simulink model "SWC_TRSP"  (R2020a)
settings: Solver=FixedStepDiscrete  StartTime=0.0  StopTime=0.15  FixedStep=0.0001  RelTol=1e-3
values from neighbouring files (symbols this model uses):
  CAL_TRSP_18VHSVoltCountTrh_s16 = 0.0    [SWC_TRSP_DataDictionary.sldd]
  CAL_TRSP_18VHSVoltDebTrh_s16 = 0.0    [SWC_TRSP_DataDictionary.sldd]
  CAL_TRSP_18VHSVoltErrRst_b = 0.0    [SWC_TRSP_DataDictionary.sldd]
  CAL_TRSP_18VHSVoltHiLim_u16 = 0.0    [SWC_TRSP_DataDictionary.sldd]
  CAL_TRSP_18VHSVoltLoLim_u16 = 0.0    [SWC_TRSP_DataDictionary.sldd]
  CAL_TRSP_1V8CPLDVoltCountTrh_s16 = 0.0    [SWC_TRSP_DataDictionary.sldd]
  CAL_TRSP_1V8CPLDVoltDebTrh_s16 = 0.0    [SWC_TRSP_DataDictionary.sldd]
  CAL_TRSP_1V8CPLDVoltErrRst_b = 0.0    [SWC_TRSP_DataDictionary.sldd]
  CAL_TRSP_1V8CPLDVoltHiLim_u16 = 0.0    [SWC_TRSP_DataDictionary.sldd]
  CAL_TRSP_1V8CPLDVoltLoLim_u16 = 0.0    [SWC_TRSP_DataDictionary.sldd]
  CAL_TRSP_3V3CPLDVoltCountTrh_s16 = 0.0    [SWC_TRSP_DataDictionary.sldd]
  CAL_TRSP_3V3CPLDVoltDebTrh_s16 = 0.0    [SWC_TRSP_DataDictionary.sldd]
  CAL_TRSP_3V3CPLDVoltErrRst_b = 0.0    [SWC_TRSP_DataDictionary.sldd]
  CAL_TRSP_3V3CPLDVoltHiLim_u16 = 0.0    [SWC_TRSP_DataDictionary.sldd]
  CAL_TRSP_3V3CPLDVoltLoLim_u16 = 0.0    [SWC_TRSP_DataDictionary.sldd]
  CAL_TRSP_AgTimecompCtl_u8 = 0.0    [SWC_TRSP_DataDictionary.sldd]
  CAL_TRSP_CurrRngCountTrh_s16 = 0.0    [SWC_TRSP_DataDictionary.sldd]
  CAL_TRSP_CurrRngDebTrh_s16 = 0.0    [SWC_TRSP_DataDictionary.sldd]
  CAL_TRSP_CurrRngErrRst_b = 0.0    [SWC_TRSP_DataDictionary.sldd]
  CAL_TRSP_CurrSumCountTrh_s16 = 0.0    [SWC_TRSP_DataDictionary.sldd]
  CAL_TRSP_CurrSumDebTrh_s16 = 0.0    [SWC_TRSP_DataDictionary.sldd]
  CAL_TRSP_CurrSumErrRst_b = 0.0    [SWC_TRSP_DataDictionary.sldd]
  CAL_TRSP_CurrSumLim_f32 = 0.0    [SWC_TRSP_DataDictionary.sldd]
  CAL_TRSP_Diff_UBR_SBCLim_f32 = 0.0    [SWC_TRSP_DataDictionary.sldd]
  CAL_TRSP_flgChangPha_b = 0.0    [SWC_TRSP_DataDictionary.sldd]
  CAL_TRSP_iPhasSensVoltCountTrh_s16 = 0.0    [SWC_TRSP_DataDictionary.sldd]
  CAL_TRSP_iPhasSensVoltDebTrh_s16 = 0.0    [SWC_TRSP_DataDictionary.sldd]
  CAL_TRSP_iPhasSensVoltErrRst_b = 0.0    [SWC_TRSP_DataDictionary.sldd]
  CAL_TRSP_iPhasSensVoltHiLim_u16 = 0.0    [SWC_TRSP_DataDictionary.sldd]
  CAL_TRSP_iPhasSensVoltLoLim_u16 = 0.0    [SWC_TRSP_DataDictionary.sldd]
  CAL_TRSP_iPhaUOffset_f32 = 0.0    [SWC_TRSP_DataDictionary.sldd]
  CAL_TRSP_iPhaVOffset_f32 = 0.0    [SWC_TRSP_DataDictionary.sldd]
  CAL_TRSP_iPhaWOffset_f32 = 0.0    [SWC_TRSP_DataDictionary.sldd]
  CAL_TRSP_iUCnvFac_f32 = 0.0    [SWC_TRSP_DataDictionary.sldd]
  CAL_TRSP_iVCnvFac_f32 = 0.0    [SWC_TRSP_DataDictionary.sldd]
  CAL_TRSP_iWCnvFac_f32 = 0.0    [SWC_TRSP_DataDictionary.sldd]
  CAL_TRSP_OfstErrRst_b = 0.0    [SWC_TRSP_DataDictionary.sldd]
  CAL_TRSP_OfstRngHiLim_f32 = 0.0    [SWC_TRSP_DataDictionary.sldd]
  CAL_TRSP_OfstRngLoLim_f32 = 0.0    [SWC_TRSP_DataDictionary.sldd]
  CAL_TRSP_ReqTrqCountTrh_s16 = 0.0    [SWC_TRSP_DataDictionary.sldd]
  CAL_TRSP_ReqTrqDebTrh_s16 = 0.0    [SWC_TRSP_DataDictionary.sldd]
  CAL_TRSP_ReqTrqErrRst_b = 0.0    [SWC_TRSP_DataDictionary.sldd]
  CAL_TRSP_ReqTrqHiLim_f32 = 0.0    [SWC_TRSP_DataDictionary.sldd]
  CAL_TRSP_ReqTrqLoLim_f32 = 0.0    [SWC_TRSP_DataDictionary.sldd]
  CAL_TRSP_RslvExciCountTrh_s16 = 0.0    [SWC_TRSP_DataDictionary.sldd]
  CAL_TRSP_RslvExciDebTrh_s16 = 0.0    [SWC_TRSP_DataDictionary.sldd]
  CAL_TRSP_RslvExciErrRst_b = 0.0    [SWC_TRSP_DataDictionary.sldd]
  CAL_TRSP_RslvMaxSele_u8 = 0.0    [SWC_TRSP_DataDictionary.sldd]
  CAL_TRSP_RslvMinSele_u8 = 0.0    [SWC_TRSP_DataDictionary.sldd]
  CAL_TRSP_RslvRngCosNHiLim_u16 = 0.0    [SWC_TRSP_DataDictionary.sldd]
  CAL_TRSP_RslvRngCosNLoLim_u16 = 0.0    [SWC_TRSP_DataDictionary.sldd]
  CAL_TRSP_RslvRngCosPHiLim_u16 = 0.0    [SWC_TRSP_DataDictionary.sldd]
  CAL_TRSP_RslvRngCosPLoLim_u16 = 0.0    [SWC_TRSP_DataDictionary.sldd]
  CAL_TRSP_RslvRngCountTrh_s16 = 0.0    [SWC_TRSP_DataDictionary.sldd]
  CAL_TRSP_RslvRngDebTrh_s16 = 0.0    [SWC_TRSP_DataDictionary.sldd]
  CAL_TRSP_RslvRngErrRst_b = 0.0    [SWC_TRSP_DataDictionary.sldd]
  CAL_TRSP_RslvRngExciHiLim_u16 = 0.0    [SWC_TRSP_DataDictionary.sldd]
  CAL_TRSP_RslvRngExciLoLim_u16 = 0.0    [SWC_TRSP_DataDictionary.sldd]
  CAL_TRSP_RslvRngSinNHiLim_u16 = 0.0    [SWC_TRSP_DataDictionary.sldd]
  CAL_TRSP_RslvRngSinNLoLim_u16 = 0.0    [SWC_TRSP_DataDictionary.sldd]
  CAL_TRSP_RslvRngSinPHiLim_u16 = 0.0    [SWC_TRSP_DataDictionary.sldd]
  CAL_TRSP_RslvRngSinPLoLim_u16 = 0.0    [SWC_TRSP_DataDictionary.sldd]
  CAL_TRSP_RslvSensVoltCountTrh_s16 = 0.0    [SWC_TRSP_DataDictionary.sldd]
  CAL_TRSP_RslvSensVoltDebTrh_s16 = 0.0    [SWC_TRSP_DataDictionary.sldd]
  CAL_TRSP_RslvSensVoltErrRst_b = 0.0    [SWC_TRSP_DataDictionary.sldd]
  CAL_TRSP_RslvSensVoltHiLim_u16 = 0.0    [SWC_TRSP_DataDictionary.sldd]
  CAL_TRSP_RslvSensVoltLoLim_u16 = 0.0    [SWC_TRSP_DataDictionary.sldd]
  CAL_TRSP_RslvSqrtCountTrh_s16 = 0.0    [SWC_TRSP_DataDictionary.sldd]
  CAL_TRSP_RslvSqrtDebTrh_s16 = 0.0    [SWC_TRSP_DataDictionary.sldd]
  CAL_TRSP_RslvSqrtErrRst_b = 0.0    [SWC_TRSP_DataDictionary.sldd]
  CAL_TRSP_RslvSqrtHiLim_u16 = 0.0    [SWC_TRSP_DataDictionary.sldd]
  CAL_TRSP_RslvSqrtLoLim_u16 = 0.0    [SWC_TRSP_DataDictionary.sldd]
  CAL_TRSP_SpeedCtlMode_u8 = 0.0    [SWC_TRSP_DataDictionary.sldd]
  CAL_TRSP_TorqueCtlMode_u8 = 0.0    [SWC_TRSP_DataDictionary.sldd]
  CAL_TRSP_UB_SBCCnvFac_f32 = 0.0    [SWC_TRSP_DataDictionary.sldd]
  CAL_TRSP_UBRVoltCountTrh_s16 = 0.0    [SWC_TRSP_DataDictionary.sldd]
  CAL_TRSP_UBRVoltDebTrh_s16 = 0.0    [SWC_TRSP_DataDictionary.sldd]
  CAL_TRSP_UBRVoltErrRst_b = 0.0    [SWC_TRSP_DataDictionary.sldd]
  CAL_TRSP_UBRWIDECnvFac_f32 = 0.0    [SWC_TRSP_DataDictionary.sldd]
  CAL_TRSP_UCurrRngHiLim_f32 = 0.0    [SWC_TRSP_DataDictionary.sldd]
  CAL_TRSP_UCurrRngLoLim_f32 = 0.0    [SWC_TRSP_DataDictionary.sldd]
  CAL_TRSP_VCurrRngHiLim_f32 = 0.0    [SWC_TRSP_DataDictionary.sldd]
  CAL_TRSP_VCurrRngLoLim_f32 = 0.0    [SWC_TRSP_DataDictionary.sldd]
  CAL_TRSP_WCurrRngHiLim_f32 = 0.0    [SWC_TRSP_DataDictionary.sldd]
  CAL_TRSP_WCurrRngLoLim_f32 = 0.0    [SWC_TRSP_DataDictionary.sldd]
  GLB_TRSP_CircAge_f32 = 0.0    [SWC_TRSP_DataDictionary.sldd]
  GLB_TRSP_MotorPole_u8 = 0.0    [SWC_TRSP_DataDictionary.sldd]
  GLB_TRSP_Sixty_f32 = 0.0    [SWC_TRSP_DataDictionary.sldd]
libraries: simulink x22
(part 1 of 13)
settings Model: DataDictionary=SWC_TRSP_DataDictionary.sldd  EnableAccessToBaseWorkspace=off  Creator=dongliyuan  LastModifiedBy=zhangjunren
settings DataIOCC: SaveFormat=StructureWithTime
settings OptimizationCC: DefaultParameterBehavior=Inlined  EnhancedBackFolding=on  PassReuseOutputArgsAs=Individual arguments  ZeroExternalMemoryAtStartup=off  ZeroInternalMemoryAtStartup=off  OptimizeBlockOrder=speed  DifferentSizesBufferReuse=on  OptimizationCustomize=off  EfficientTunableParamExpr=on
settings DebuggingCC: SignalInfNanChecking=warning  ParameterPrecisionLossMsg=none  ParameterTunabilityLossMsg=error  UnnecessaryDatatypeConvMsg=warning  VectorMatrixConversionMsg=warning  StrictBusMsg=WarnOnBusTreatedAsVector  NonBusSignalsTreatedAsBus=warning
settings ModelReferenceCC: ModelReferenceNumInstancesAllowed=Single
settings SFSimCC: MATLABDynamicMemAlloc=off
settings RTWCC: SystemTargetFile=ert.tlc  GenCodeOnly=on  TemplateMakefile=ert_default_tmf  CustomSourceCode="#include \"set_get_data.h\""
settings CodeAppCC: ForceParamTrailComments=on  IgnoreCustomStorageClasses=off  OperatorAnnotations=on  SimulinkDataObjDesc=on  SFDataObjDesc=on  InsertBlockDesc=on
settings ERTTargetCC: TargetLangStandard=C99 (ISO)  UtilityFuncGeneration=Shared location  IncludeMdlTerminateFcn=off  GenerateASAP2=on  InlinedParameterPlacement=NonHierarchical  ERTCustomFileTemplate=example_file_process.tlc  EnableUserReplacementTypes=on

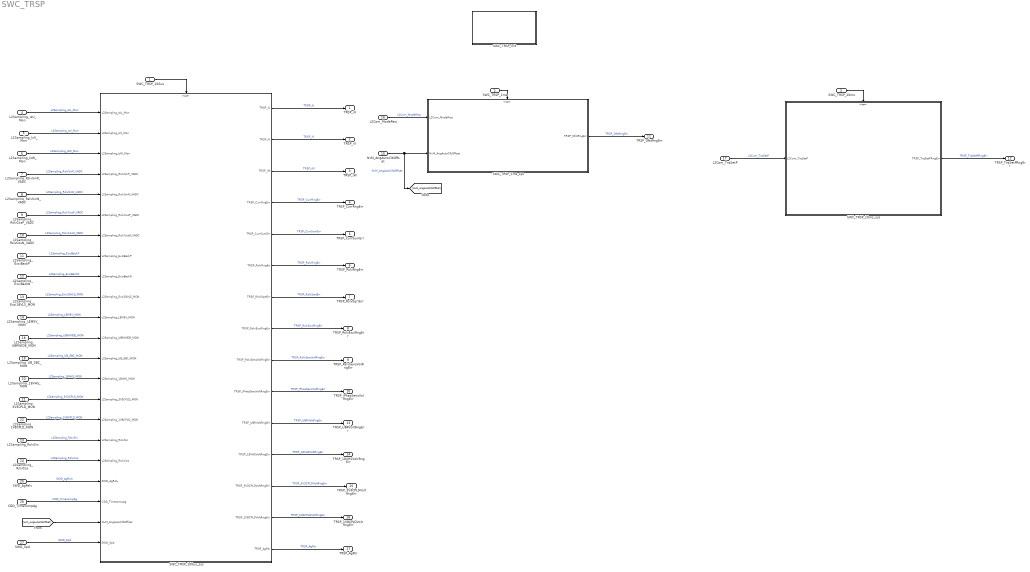
== system SWC_TRSP ==
  SWC_TRSP_100us : Inport  SampleTime=0.0001  OutputFunctionCall=on
  SWC_TRSP_1ms : Inport  Port=2  SampleTime=0.001  OutputFunctionCall=on
  SWC_TRSP_10ms : Inport  Port=3  SampleTime=0.01  OutputFunctionCall=on
  L2Sampling_IsU_Mon : Inport  Port=4
  L2Sampling_IsV_Mon : Inport  Port=5
  L2Sampling_IsW_Mon : Inport  Port=6
  L2Sampling_RslvSinP_VADC : Inport  Port=7  PortDimensions=[1 32]
  L2Sampling_RslvSinN_VADC : Inport  Port=8  PortDimensions=[1 32]
  L2Sampling_RslvCosP_VADC : Inport  Port=9  PortDimensions=[1 32]
  L2Sampling_RslvCosN_VADC : Inport  Port=10
  L2Sampling_ExciBackP : Inport  Port=11
  L2Sampling_ExciBackN : Inport  Port=12
  L2Sampling_Exci18VLS_MON : Inport  Port=13
  L2Sampling_LEM5V_MON : Inport  Port=14
  NvM_AngAutoClbOffset : Inport  Port=15
  L2Com_ModeReq : Inport  Port=16  PortDimensions=1
  L2Com_TrqSetP : Inport  Port=17  PortDimensions=1
  L2Sampling_UBRWIDE_MON : Inport  Port=18
  L2Sampling_UB_SBC_MON : Inport  Port=19
  L2Sampling_18VHS_MON : Inport  Port=20
  L2Sampling_3V3CPLD_MON : Inport  Port=21
  L2Sampling_1V8CPLD_MON : Inport  Port=22
  L2Sampling_RslvSin : Inport  Port=23
  L2Sampling_RslvCos : Inport  Port=24
  SWD_AgRslv : Inport  Port=25
  CDD_TimecompAg : Inport  Port=26
  SWD_Spd : Inport  Port=27
  SWC_TRSP_100us_sys : Subsystem
  SWC_TRSP_10ms_sys : Subsystem
  SWC_TRSP_1ms_sys : Subsystem
  SWC_TRSP_Init : Subsystem
  TRSP_iU : Outport
  TRSP_iV : Outport  Port=2
  TRSP_iW : Outport  Port=3
  TRSP_CurrRngErr : Outport  Port=4
  TRSP_CurrSumErr : Outport  Port=5
  TRSP_RslvRngErr : Outport  Port=6
  TRSP_RslvSqrtErr : Outport  Port=7
  TRSP_RslvExciRngErr : Outport  Port=8
  TRSP_RslvSensVolRngErr : Outport  Port=9
  TRSP_iPhasSensVolRngErr : Outport  Port=10
  TRSP_OfstRngErr : Outport  Port=11
  TRSP_TrqSetPRngErr : Outport  Port=12
  TRSP_UBRVoltRngErr : Outport  Port=13
  TRSP_18VHSVoltRngErr : Outport  Port=14
  TRSP_3V3CPLDVoltRngErr : Outport  Port=15
  TRSP_1V8CPLDVoltRngErr : Outport  Port=16
  TRSP_AgRtr : Outport  Port=17
  wires:
  SWC_TRSP_100us_sys/10(TRSP_iPhasSensVoltRngErr) -> TRSP_iPhasSensVolRngErr/1  "TRSP_iPhasSensVolRngErr"
  L2Sampling_IsU_Mon/1 -> SWC_TRSP_100us_sys/1(L2Sampling_IsU_Mon)  "L2Sampling_IsU_Mon"
  L2Sampling_LEM5V_MON/1 -> SWC_TRSP_100us_sys/11(L2Sampling_LEM5V_MON)  "L2Sampling_LEM5V_MON"
  L2Sampling_IsV_Mon/1 -> SWC_TRSP_100us_sys/2(L2Sampling_IsV_Mon)  "L2Sampling_IsV_Mon"
  L2Sampling_ExciBackN/1 -> SWC_TRSP_100us_sys/9(L2Sampling_ExciBackN)  "L2Sampling_ExciBackN"
  L2Sampling_ExciBackP/1 -> SWC_TRSP_100us_sys/8(L2Sampling_ExciBackP)  "L2Sampling_ExciBackP"
  L2Sampling_Exci18VLS_MON/1 -> SWC_TRSP_100us_sys/10(L2Sampling_Exci18VLS_MON)  "L2Sampling_Exci18VLS_MON"
  SWC_TRSP_1ms_sys/1(TRSP_OfstRngErr) -> TRSP_OfstRngErr/1  "TRSP_OfstRngErr"
  L2Sampling_RslvCosP_VADC/1 -> SWC_TRSP_100us_sys/6(L2Sampling_RslvCosP_VADC)  "L2Sampling_RslvCosP_VADC"
  SWC_TRSP_100us_sys/4(TRSP_CurrRngErr) -> TRSP_CurrRngErr/1  "TRSP_CurrRngErr"
  NvM_AngAutoClbOffset/1 -> SWC_TRSP_1ms_sys/2(NvM_AngAutoClbOffset), [NvM_AngAutoClbOffset]  "NvM_AngAutoClbOffset"
  SWC_TRSP_100us_sys/7(TRSP_RslvSqrtErr) -> TRSP_RslvSqrtErr/1  "TRSP_RslvSqrtErr"
  SWC_TRSP_100us_sys/3(TRSP_iW) -> TRSP_iW/1  "TRSP_iW"
  L2Sampling_RslvSinP_VADC/1 -> SWC_TRSP_100us_sys/4(L2Sampling_RslvSinP_VADC)  "L2Sampling_RslvSinP_VADC"
  L2Sampling_IsW_Mon/1 -> SWC_TRSP_100us_sys/3(L2Sampling_IsW_Mon)  "L2Sampling_IsW_Mon"
  SWC_TRSP_100us_sys/9(TRSP_RslvSensVolRngErr) -> TRSP_RslvSensVolRngErr/1  "TRSP_RslvSensVolRngErr"
  SWC_TRSP_100us_sys/2(TRSP_iV) -> TRSP_iV/1  "TRSP_iV"
  SWC_TRSP_100us_sys/1(TRSP_iU) -> TRSP_iU/1  "TRSP_iU"
  SWC_TRSP_100us_sys/5(TRSP_CurrSumErr) -> TRSP_CurrSumErr/1  "TRSP_CurrSumErr"
  SWC_TRSP_100us_sys/8(TRSP_RslvExciRngErr) -> TRSP_RslvExciRngErr/1  "TRSP_RslvExciRngErr"
  SWC_TRSP_100us_sys/6(TRSP_RslvRngErr) -> TRSP_RslvRngErr/1  "TRSP_RslvRngErr"
  SWC_TRSP_100us/1 -> SWC_TRSP_100us_sys/Trigger
  SWC_TRSP_1ms/1 -> SWC_TRSP_1ms_sys/Trigger
  L2Com_TrqSetP/1 -> SWC_TRSP_10ms_sys/1(L2Com_TrqSetP)  "L2Com_TrqSetP"
  SWC_TRSP_10ms_sys/1(TRSP_TrqSetPRngErr) -> TRSP_TrqSetPRngErr/1  "TRSP_TrqSetPRngErr"
  L2Sampling_RslvSinN_VADC/1 -> SWC_TRSP_100us_sys/5(L2Sampling_RslvSinN_VADC)  "L2Sampling_RslvSinN_VADC"
  L2Sampling_RslvCosN_VADC/1 -> SWC_TRSP_100us_sys/7(L2Sampling_RslvCosN_VADC)  "L2Sampling_RslvCosN_VADC"
  SWC_TRSP_10ms/1 -> SWC_TRSP_10ms_sys/Trigger
  L2Com_ModeReq/1 -> SWC_TRSP_1ms_sys/1(L2Com_ModeReq)  "L2Com_ModeReq"
  L2Sampling_1V8CPLD_MON/1 -> SWC_TRSP_100us_sys/16(L2Sampling_1V8CPLD_MON)  "L2Sampling_1V8CPLD_MON"
  L2Sampling_UB_SBC_MON/1 -> SWC_TRSP_100us_sys/13(L2Sampling_UB_SBC_MON)  "L2Sampling_UB_SBC_MON"
  L2Sampling_3V3CPLD_MON/1 -> SWC_TRSP_100us_sys/15(L2Sampling_3V3CPLD_MON)  "L2Sampling_3V3CPLD_MON"
  L2Sampling_UBRWIDE_MON/1 -> SWC_TRSP_100us_sys/12(L2Sampling_UBRWIDE_MON)  "L2Sampling_UBRWIDE_MON"
  L2Sampling_18VHS_MON/1 -> SWC_TRSP_100us_sys/14(L2Sampling_18VHS_MON)  "L2Sampling_18VHS_MON"
  SWC_TRSP_100us_sys/14(TRSP_1V8CPLDVoltRngErr) -> TRSP_1V8CPLDVoltRngErr/1  "TRSP_1V8CPLDVoltRngErr"
  SWC_TRSP_100us_sys/12(TRSP_18VHSVoltRngErr) -> TRSP_18VHSVoltRngErr/1  "TRSP_18VHSVoltRngErr"
  SWC_TRSP_100us_sys/11(TRSP_UBRVoltRngErr) -> TRSP_UBRVoltRngErr/1  "TRSP_UBRVoltRngErr"
  SWC_TRSP_100us_sys/13(TRSP_3V3CPLDVoltRngErr) -> TRSP_3V3CPLDVoltRngErr/1  "TRSP_3V3CPLDVoltRngErr"
  L2Sampling_RslvSin/1 -> SWC_TRSP_100us_sys/17(L2Sampling_RslvSin)  "L2Sampling_RslvSin"
  L2Sampling_RslvCos/1 -> SWC_TRSP_100us_sys/18(L2Sampling_RslvCos)  "L2Sampling_RslvCos"
  SWD_AgRslv/1 -> SWC_TRSP_100us_sys/19(SWD_AgRslv)  "SWD_AgRslv"
  CDD_TimecompAg/1 -> SWC_TRSP_100us_sys/20(CDD_TimecompAg)  "CDD_TimecompAg"
  SWD_Spd/1 -> SWC_TRSP_100us_sys/22(SWD_Spd)  "SWD_Spd"
  [NvM_AngAutoClbOffset] -> SWC_TRSP_100us_sys/21(NvM_AngAutoClbOffset)
  SWC_TRSP_100us_sys/15(TRSP_AgRtr) -> TRSP_AgRtr/1  "TRSP_AgRtr"
